simulink model "sim3el17128"  (R2019b)
settings: Solver=ode45  StartTime=0.0  StopTime=10  MaxStep=1e-4  RelTol=1e-4
values from neighbouring files (symbols this model uses):
  b1 = 0.1796    [scriptsim3el17128.m]
  b2 = 0.0012    [scriptsim3el17128.m]
  Idref = psi_hat/LM    (= 5.01212611156)    [scriptsim3el17128.m]
  Iqref = sqrt(Iref^2-Idref^2)    [scriptsim3el17128.m]
  J = 0.08    [scriptsim3el17128.m]
  K = 1/sqrt(2)    [scriptsim3el17128.m]
  Ki = alphaC*(R+Ra)    [scriptsim3el17128.m]
  kip = alphaP*alphaP/psi_hat    (= 19516.1290323)    [scriptsim3el17128.m]
  Kp = alphaC*L    [scriptsim3el17128.m]
  kpp = 2*alphaP/psi_hat    (= 354.838709677)    [scriptsim3el17128.m]
  L = Lsigma    (= 0.0227)    [scriptsim3el17128.m]
  LM = 0.1237    [scriptsim3el17128.m]
  Lsigma = 0.0227    [scriptsim3el17128.m]
  np = 2    [scriptsim3el17128.m]
  phi_a = 0    [scriptsim3el17128.m]
  phi_b = -2*pi/3    (= -2.09439510239)    [scriptsim3el17128.m]
  phi_c = -4*pi/3    (= -4.18879020479)    [scriptsim3el17128.m]
  psi_hat = 0.62    [scriptsim3el17128.m]
  Ra = alphaC*L - R    [scriptsim3el17128.m]
  refsw = 0    [scriptsim3el17128.m]
  RR = 0.8197    [scriptsim3el17128.m]
  Rs = 2.2667    [scriptsim3el17128.m]
  sw1 = 1    [scriptsim3el17128.m]
  sw2 = 1    [scriptsim3el17128.m]
  sw3 = 1    [scriptsim3el17128.m]
  tL = 26.8    [scriptsim3el17128.m]
  Vhat = 230*sqrt(2)    [scriptsim3el17128.m]
  w = 2*pi*f    (= 314.159265359)    [scriptsim3el17128.m]
undefined symbols (not defined in the file or in its folder): magnitude
settings Model: DataTypeOverride=Double  MinMaxOverflowLogging=ForceOff  Creator=user  LastModifiedBy=user
settings SolverCC: ZeroCrossAlgorithm=Adaptive
settings DebuggingCC: IgnoredZcDiagnostic=none

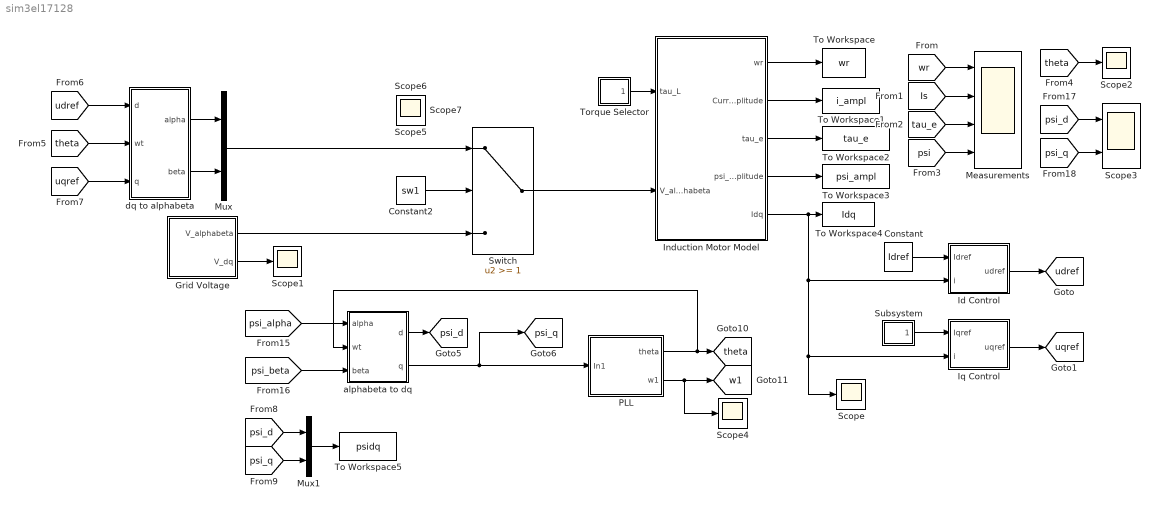
== system sim3el17128 ==
  Constant : Constant  Value=Idref
  Constant2 : Constant  Value=sw1
  Grid Voltage : Subsystem
  Id Control : Subsystem
  Induction Motor Model : Subsystem
  Iq Control : Subsystem
  Measurements : Scope  NumInputPorts=4
  Mux : Mux  Inputs=2
  Mux1 : Mux  Inputs=2
  PLL : Subsystem
  Scope{,1..2,4..7} (7 alike) : Scope
  Scope3 : Scope  NumInputPorts=2
  Subsystem : Subsystem
  Switch : Switch  Threshold=1
  To Workspace : ToWorkspace  VariableName=wr  SaveFormat=Timeseries  SampleTime=-1
  To Workspace1 : ToWorkspace  VariableName=i_ampl  SaveFormat=Timeseries  SampleTime=-1
  To Workspace2 : ToWorkspace  VariableName=tau_e  SaveFormat=Timeseries  SampleTime=-1
  To Workspace3 : ToWorkspace  VariableName=psi_ampl  SaveFormat=Timeseries  SampleTime=-1
  To Workspace4 : ToWorkspace  VariableName=Idq  SaveFormat=Timeseries  SampleTime=-1
  To Workspace5 : ToWorkspace  VariableName=psidq  SaveFormat=Timeseries  SampleTime=-1
  Torque Selector : Subsystem
  alphabeta to dq : Subsystem
  dq to alphabeta : Subsystem
  tag scope: psi_d=global, psi_q=global, theta=global, udref=global, uqref=global, w1=global
  wires:
  Induction Motor Model/1(wr) -> To Workspace/1
  Induction Motor Model/3(tau_e) -> To Workspace2/1
  Induction Motor Model/2(Current amplitude) -> To Workspace1/1
  Induction Motor Model/4(psi_amplitude) -> To Workspace3/1
  [wr] -> Measurements/1
  [Is] -> Measurements/2
  [tau_e] -> Measurements/3
  [psi] -> Measurements/4
  [theta] -> Scope2/1
  [theta] -> dq to alphabeta/2(wt)
  dq to alphabeta/1(alpha) -> Mux/1
  dq to alphabeta/2(beta) -> Mux/2
  [psi_q] -> Scope3/2
  [psi_d] -> Scope3/1
  PLL/1(theta) -> alphabeta to dq/2(wt), [theta]
  alphabeta to dq/2(q) -> [psi_q], PLL/1(In1)
  [psi_alpha] -> alphabeta to dq/1(alpha)
  PLL/2(w1) -> Scope4/1, [w1]
  [psi_beta] -> alphabeta to dq/3(beta)
  alphabeta to dq/1(d) -> [psi_d]
  [udref] -> dq to alphabeta/1(d)
  [uqref] -> dq to alphabeta/3(q)
  Induction Motor Model/5(Idq) -> To Workspace4/1, Id Control/2(i), Scope/1, Iq Control/2(i)
  Iq Control/1(uqref) -> [uqref]
  Constant/1 -> Id Control/1(Idref)
  Id Control/1(udref) -> [udref]
  Torque Selector/1(tau_L) -> Induction Motor Model/1(tau_L)
  Switch/1 -> Induction Motor Model/2(V_alphabeta)
  Grid Voltage/1(V_alphabeta) -> Switch/3
  Constant2/1 -> Switch/2
  Mux/1 -> Switch/1
  Grid Voltage/2(V_dq) -> Scope1/1
  [psi_q] -> Mux1/2
  [psi_d] -> Mux1/1
  Mux1/1 -> To Workspace5/1
  Subsystem/1(Iqref) -> Iq Control/1(Iqref)

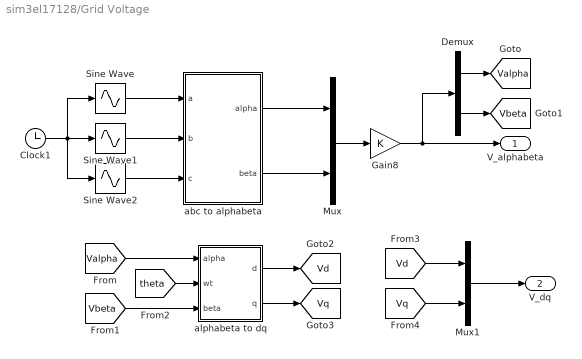
== system sim3el17128/Grid Voltage ==
  Clock1 : Clock
  Demux : Demux  Outputs=2
  Gain8 : Gain  Gain=K
  Mux : Mux  Inputs=2
  Mux1 : Mux  Inputs=2
  Sine Wave : Sin  TimeSource=Use external signal  Amplitude=Vhat  Frequency=w  Phase=phi_a  SampleTime=0
  Sine Wave1 : Sin  TimeSource=Use external signal  Amplitude=Vhat  Frequency=w  Phase=phi_b  SampleTime=0
  Sine Wave2 : Sin  TimeSource=Use external signal  Amplitude=Vhat  Frequency=w  Phase=phi_c  SampleTime=0
  abc to alphabeta : Subsystem
  alphabeta to dq : Subsystem
  V_alphabeta : Outport
  V_dq : Outport  Port=2
  tag scope: Valpha=global, Vbeta=global, Vd=global, Vq=global
  wires:
  Clock1/1 -> Sine Wave1/1, Sine Wave2/1, Sine Wave/1
  Mux/1 -> Gain8/1
  Gain8/1 -> Demux/1, V_alphabeta/1
  Demux/2 -> [Vbeta]
  Demux/1 -> [Valpha]
  [Valpha] -> alphabeta to dq/1(alpha)
  [Vbeta] -> alphabeta to dq/3(beta)
  [theta] -> alphabeta to dq/2(wt)
  alphabeta to dq/1(d) -> [Vd]
  alphabeta to dq/2(q) -> [Vq]
  [Vq] -> Mux1/2
  [Vd] -> Mux1/1
  Mux1/1 -> V_dq/1
  Sine Wave/1 -> abc to alphabeta/1(a)
  Sine Wave1/1 -> abc to alphabeta/2(b)
  Sine Wave2/1 -> abc to alphabeta/3(c)
  abc to alphabeta/1(alpha) -> Mux/1
  abc to alphabeta/2(beta) -> Mux/2

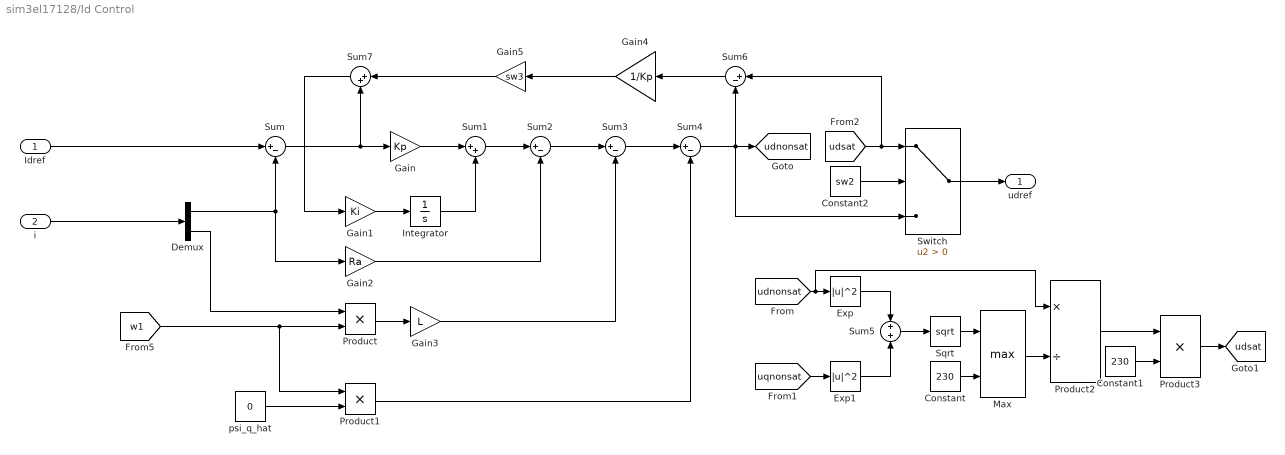
== system sim3el17128/Id Control ==
  Idref : Inport
  i : Inport  Port=2
  Constant : Constant  Value=230
  Constant1 : Constant  Value=230
  Constant2 : Constant  Value=sw2
  Demux : Demux  Outputs=2
  Exp : Math  Operator=magnitude^2  SignedPower=off  SaturateOnIntegerOverflow=on
  Exp1 : Math  Operator=magnitude^2  SignedPower=off  SaturateOnIntegerOverflow=on
  Gain : Gain  Gain=Kp
  Gain1 : Gain  Gain=Ki
  Gain2 : Gain  Gain=Ra
  Gain3 : Gain  Gain=L
  Gain4 : Gain  Gain=1/Kp
  Gain5 : Gain  Gain=sw3
  Integrator : Integrator
  Max : MinMax  Function=max  Inputs=2
  Product : Product
  Product1 : Product
  Product2 : Product  Inputs=*/
  Product3 : Product
  Sqrt : Sqrt  SaturateOnIntegerOverflow=on
  Sum{,2..4,6} (5 alike) : Sum  Inputs=|+-
  Sum1 : Sum  Inputs=|++
  Sum5 : Sum
  Sum7 : Sum  Inputs=|++
  Switch : Switch  Criteria=u2 > Threshold
  psi_q_hat : Constant  Value=0
  udref : Outport
  tag scope: udnonsat=global, udsat=global
  wires:
  Sum/1 -> Sum7/2, Gain/1
  Product1/1 -> Sum4/2
  psi_q_hat/1 -> Product1/2
  Demux/2 -> Product/1
  Sum3/1 -> Sum4/1
  Gain2/1 -> Sum2/2
  Demux/1 -> Gain2/1, Sum/2
  Gain/1 -> Sum1/1
  Sum2/1 -> Sum3/1
  Sum1/1 -> Sum2/1
  Gain3/1 -> Sum3/2
  Gain1/1 -> Integrator/1
  Product/1 -> Gain3/1
  Integrator/1 -> Sum1/2
  i/1 -> Demux/1
  Idref/1 -> Sum/1
  [udnonsat] -> Product2/1, Exp/1
  [uqnonsat] -> Exp1/1
  Exp/1 -> Sum5/1
  Exp1/1 -> Sum5/2
  Sum5/1 -> Sqrt/1
  Sqrt/1 -> Max/1
  Constant/1 -> Max/2
  Max/1 -> Product2/2
  Product2/1 -> Product3/1
  Constant1/1 -> Product3/2
  Product3/1 -> [udsat]
  [udsat] -> Switch/1, Sum6/1
  Sum7/1 -> Gain1/1
  Gain4/1 -> Gain5/1
  Sum6/1 -> Gain4/1
  [w1] -> Product1/1, Product/2
  Switch/1 -> udref/1
  Constant2/1 -> Switch/2
  Gain5/1 -> Sum7/1
  Sum4/1 -> Switch/3, Sum6/2, [udnonsat]

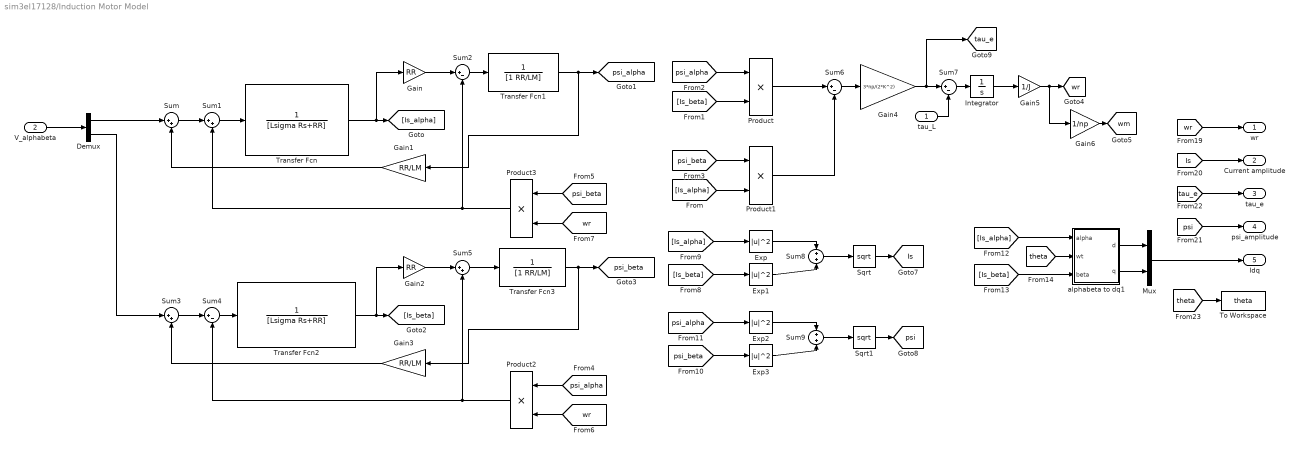
== system sim3el17128/Induction Motor Model ==
  tau_L : Inport
  V_alphabeta : Inport  Port=2
  Demux : Demux  Outputs=2
  Exp{,1..3} (4 alike) : Math  Operator=magnitude^2  SignedPower=off  SaturateOnIntegerOverflow=on
  Gain : Gain  Gain=RR
  Gain1 : Gain  Gain=RR/LM
  Gain2 : Gain  Gain=RR
  Gain3 : Gain  Gain=RR/LM
  Gain4 : Gain  Gain=3*np/(2*K^2)
  Gain5 : Gain  Gain=1/J
  Gain6 : Gain  Gain=1/np
  Integrator : Integrator
  Mux : Mux  Inputs=2
  Product{,1..3} (4 alike) : Product
  Sqrt : Sqrt  SaturateOnIntegerOverflow=on
  Sqrt1 : Sqrt  SaturateOnIntegerOverflow=on
  Sum{,1,3,5} (4 alike) : Sum  Inputs=|++
  Sum{2,4,6..7} (4 alike) : Sum  Inputs=|+-
  Sum8 : Sum  Inputs=+|+
  Sum9 : Sum  Inputs=+|+
  To Workspace : ToWorkspace  VariableName=theta  SaveFormat=Timeseries  SampleTime=-1
  Transfer Fcn : TransferFcn  Denominator=[Lsigma Rs+RR]
  Transfer Fcn1 : TransferFcn  Denominator=[1 RR/LM]
  Transfer Fcn2 : TransferFcn  Denominator=[Lsigma Rs+RR]
  Transfer Fcn3 : TransferFcn  Denominator=[1 RR/LM]
  alphabeta to dq1 : Subsystem
  wr : Outport
  Current amplitude : Outport  Port=2
  tau_e : Outport  Port=3
  psi_amplitude : Outport  Port=4
  Idq : Outport  Port=5
  tag scope: Is=global, psi=global, psi_alpha=global, psi_beta=global, tau_e=global, wm=global, wr=global
  wires:
  Transfer Fcn1/1 -> Gain1/1, [psi_alpha]
  Product3/1 -> Sum1/2, Sum2/2
  Product2/1 -> Sum4/2, Sum5/2
  [Is_beta] -> Exp1/1
  Gain5/1 -> Gain6/1, [wr]
  [Is_beta] -> Product/2
  Product/1 -> Sum6/1
  [wr] -> Product2/2
  Sqrt/1 -> [Is]
  Sum3/1 -> Sum4/1
  Transfer Fcn3/1 -> Gain3/1, [psi_beta]
  [psi_beta] -> Product1/1
  Sum5/1 -> Transfer Fcn3/1
  Transfer Fcn2/1 -> Gain2/1, [Is_beta]
  Sum1/1 -> Transfer Fcn/1
  V_alphabeta/1 -> Demux/1
  [Is_alpha] -> Product1/2
  Gain1/1 -> Sum/2
  Demux/2 -> Sum3/1
  Demux/1 -> Sum/1
  Exp/1 -> Sum8/1
  tau_L/1 -> Sum7/2
  Sum/1 -> Sum1/1
  Sum6/1 -> Gain4/1
  Gain4/1 -> [tau_e], Sum7/1
  Transfer Fcn/1 -> Gain/1, [Is_alpha]
  [psi_alpha] -> Product/1
  Sum2/1 -> Transfer Fcn1/1
  Gain3/1 -> Sum3/2
  Gain2/1 -> Sum5/1
  Sum4/1 -> Transfer Fcn2/1
  Product1/1 -> Sum6/2
  [Is_alpha] -> Exp/1
  Sum8/1 -> Sqrt/1
  Gain/1 -> Sum2/1
  [wr] -> Product3/2
  [psi_beta] -> Product3/1
  Sum7/1 -> Integrator/1
  Integrator/1 -> Gain5/1
  [psi_alpha] -> Product2/1
  Exp1/1 -> Sum8/2
  Sum9/1 -> Sqrt1/1
  [psi_alpha] -> Exp2/1
  Exp3/1 -> Sum9/2
  [psi_beta] -> Exp3/1
  Exp2/1 -> Sum9/1
  Sqrt1/1 -> [psi]
  Mux/1 -> Idq/1
  alphabeta to dq1/2(q) -> Mux/2
  alphabeta to dq1/1(d) -> Mux/1
  [Is_beta] -> alphabeta to dq1/3(beta)
  [Is_alpha] -> alphabeta to dq1/1(alpha)
  [theta] -> alphabeta to dq1/2(wt)
  [wr] -> wr/1
  [Is] -> Current amplitude/1
  [psi] -> psi_amplitude/1
  [tau_e] -> tau_e/1
  [theta] -> To Workspace/1
  Gain6/1 -> [wm]

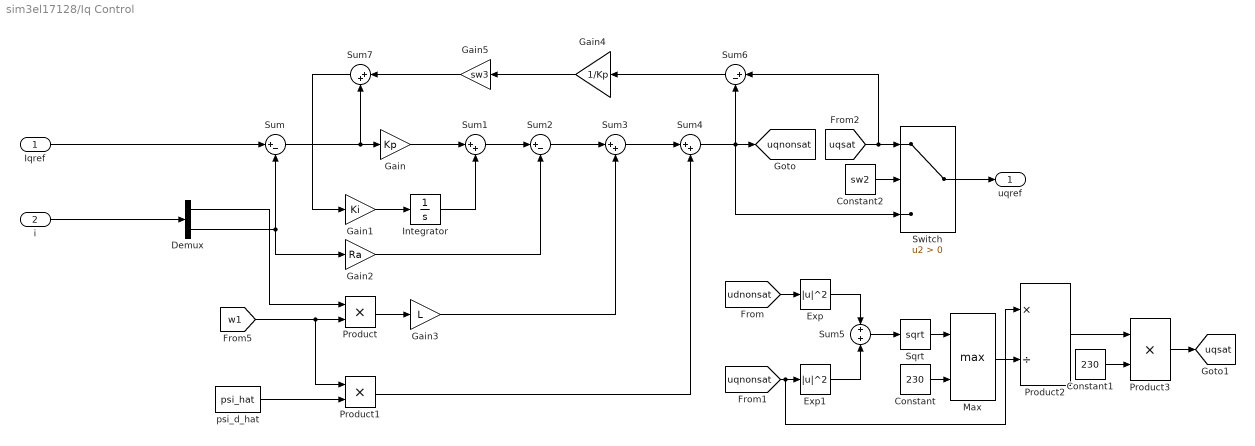
== system sim3el17128/Iq Control ==
  Iqref : Inport
  i : Inport  Port=2
  Constant : Constant  Value=230
  Constant1 : Constant  Value=230
  Constant2 : Constant  Value=sw2
  Demux : Demux  Outputs=2
  Exp : Math  Operator=magnitude^2  SignedPower=off  SaturateOnIntegerOverflow=on
  Exp1 : Math  Operator=magnitude^2  SignedPower=off  SaturateOnIntegerOverflow=on
  Gain : Gain  Gain=Kp
  Gain1 : Gain  Gain=Ki
  Gain2 : Gain  Gain=Ra
  Gain3 : Gain  Gain=L
  Gain4 : Gain  Gain=1/Kp
  Gain5 : Gain  Gain=sw3
  Integrator : Integrator
  Max : MinMax  Function=max  Inputs=2
  Product : Product
  Product1 : Product
  Product2 : Product  Inputs=*/
  Product3 : Product
  Sqrt : Sqrt  SaturateOnIntegerOverflow=on
  Sum : Sum  Inputs=|+-
  Sum{1,3..4,7} (4 alike) : Sum  Inputs=|++
  Sum2 : Sum  Inputs=|+-
  Sum5 : Sum
  Sum6 : Sum  Inputs=|+-
  Switch : Switch  Criteria=u2 > Threshold
  psi_d_hat : Constant  Value=psi_hat
  uqref : Outport
  tag scope: uqnonsat=global, uqsat=global
  wires:
  Iqref/1 -> Sum/1
  i/1 -> Demux/1
  Integrator/1 -> Sum1/2
  Product/1 -> Gain3/1
  Gain1/1 -> Integrator/1
  Gain3/1 -> Sum3/2
  Sum1/1 -> Sum2/1
  Sum2/1 -> Sum3/1
  Gain/1 -> Sum1/1
  Gain2/1 -> Sum2/2
  Sum3/1 -> Sum4/1
  psi_d_hat/1 -> Product1/2
  Product1/1 -> Sum4/2
  [w1] -> Product/2, Product1/1
  Demux/2 -> Sum/2, Gain2/1
  Demux/1 -> Product/1
  Sum/1 -> Sum7/2, Gain/1
  Exp1/1 -> Sum5/2
  Constant1/1 -> Product3/2
  Max/1 -> Product2/2
  Sum5/1 -> Sqrt/1
  Constant/1 -> Max/2
  Product3/1 -> [uqsat]
  Sqrt/1 -> Max/1
  Product2/1 -> Product3/1
  [uqnonsat] -> Product2/1, Exp1/1
  Exp/1 -> Sum5/1
  [udnonsat] -> Exp/1
  Sum6/1 -> Gain4/1
  Gain4/1 -> Gain5/1
  Sum7/1 -> Gain1/1
  [uqsat] -> Sum6/1, Switch/1
  Switch/1 -> uqref/1
  Constant2/1 -> Switch/2
  Gain5/1 -> Sum7/1
  Sum4/1 -> Switch/3, Sum6/2, [uqnonsat]

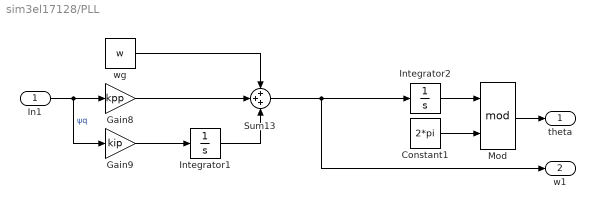
== system sim3el17128/PLL ==
  In1 : Inport
  Constant1 : Constant  Value=2*pi
  Gain8 : Gain  Gain=kpp
  Gain9 : Gain  Gain=kip
  Integrator1 : Integrator
  Integrator2 : Integrator
  Mod : Math  Operator=mod  SignedPower=off  SaturateOnIntegerOverflow=on
  Sum13 : Sum  Inputs=+++
  wg : Constant  Value=w
  theta : Outport
  w1 : Outport  Port=2
  wires:
  In1/1 -> Gain9/1, Gain8/1  "ψq"
  Constant1/1 -> Mod/2
  Gain8/1 -> Sum13/2
  wg/1 -> Sum13/1
  Gain9/1 -> Integrator1/1
  Integrator1/1 -> Sum13/3
  Sum13/1 -> w1/1, Integrator2/1
  Mod/1 -> theta/1
  Integrator2/1 -> Mod/1

== system sim3el17128/Subsystem ==
  Constant1 : Constant  Value=Iqref
  Constant2 : Constant  Value=0
  Constant3 : Constant  Value=refsw
  Constant4 : Constant  Value=Iqref
  Switch1 : Switch  Threshold=w
  Switch2 : Switch  Criteria=u2 > Threshold
  Iqref : Outport
  wires:
  Constant2/1 -> Switch1/1
  Constant1/1 -> Switch1/3
  [wr] -> Switch1/2
  Switch1/1 -> Switch2/1
  Constant4/1 -> Switch2/3
  Switch2/1 -> Iqref/1
  Constant3/1 -> Switch2/2

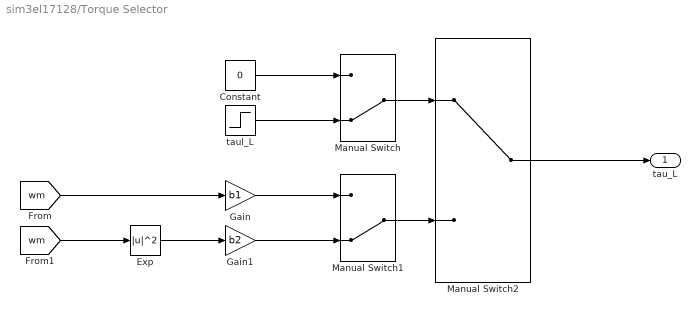
== system sim3el17128/Torque Selector ==
  Constant : Constant  Value=0
  Exp : Math  Operator=magnitude^2  SignedPower=off  SaturateOnIntegerOverflow=on
  Gain : Gain  Gain=b1
  Gain1 : Gain  Gain=b2
  Manual Switch : ManualSwitch  CurrentSetting=0
  Manual Switch1 : ManualSwitch  CurrentSetting=0
  Manual Switch2 : ManualSwitch
  taul_L : Step  Time=5  After=tL  SampleTime=0
  tau_L : Outport
  wires:
  [wm] -> Gain/1
  Gain1/1 -> Manual Switch1/2
  taul_L/1 -> Manual Switch/2
  Exp/1 -> Gain1/1
  [wm] -> Exp/1
  Constant/1 -> Manual Switch/1
  Gain/1 -> Manual Switch1/1
  Manual Switch2/1 -> tau_L/1
  Manual Switch1/1 -> Manual Switch2/2
  Manual Switch/1 -> Manual Switch2/1

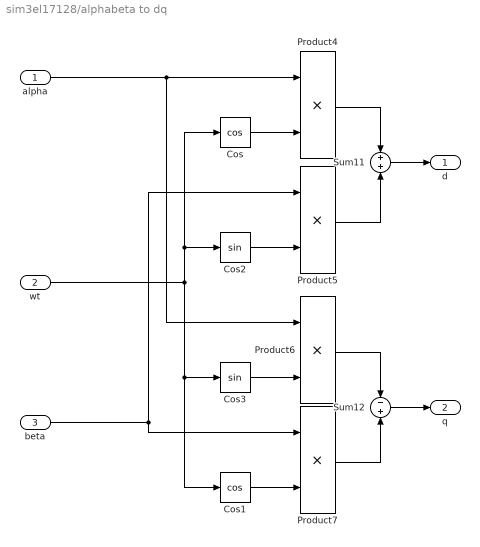
== system sim3el17128/alphabeta to dq ==
  alpha : Inport
  wt : Inport  Port=2
  beta : Inport  Port=3
  Cos : Trigonometry  Operator=cos
  Cos1 : Trigonometry  Operator=cos
  Cos2 : Trigonometry
  Cos3 : Trigonometry
  Product{4..7} (4 alike) : Product
  Sum11 : Sum
  Sum12 : Sum  Inputs=-+
  d : Outport
  q : Outport  Port=2
  wires:
  Cos3/1 -> Product6/2
  Product6/1 -> Sum12/1
  Sum11/1 -> d/1
  alpha/1 -> Product4/1, Product6/1
  wt/1 -> Cos3/1, Cos1/1, Cos2/1, Cos/1
  Product4/1 -> Sum11/1
  beta/1 -> Product7/1, Product5/1
  Product7/1 -> Sum12/2
  Cos1/1 -> Product7/2
  Product5/1 -> Sum11/2
  Cos/1 -> Product4/2
  Cos2/1 -> Product5/2
  Sum12/1 -> q/1

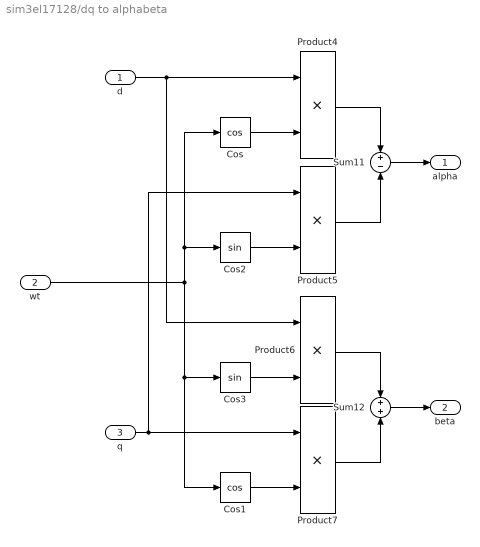
== system sim3el17128/dq to alphabeta ==
  d : Inport
  wt : Inport  Port=2
  q : Inport  Port=3
  Cos : Trigonometry  Operator=cos
  Cos1 : Trigonometry  Operator=cos
  Cos2 : Trigonometry
  Cos3 : Trigonometry
  Product{4..7} (4 alike) : Product
  Sum11 : Sum  Inputs=+-
  Sum12 : Sum
  alpha : Outport
  beta : Outport  Port=2
  wires:
  Cos3/1 -> Product6/2
  Product6/1 -> Sum12/1
  Sum11/1 -> alpha/1
  d/1 -> Product4/1, Product6/1
  wt/1 -> Cos3/1, Cos1/1, Cos2/1, Cos/1
  Product4/1 -> Sum11/1
  q/1 -> Product5/1, Product7/1
  Product7/1 -> Sum12/2
  Cos1/1 -> Product7/2
  Product5/1 -> Sum11/2
  Cos/1 -> Product4/2
  Cos2/1 -> Product5/2
  Sum12/1 -> beta/1

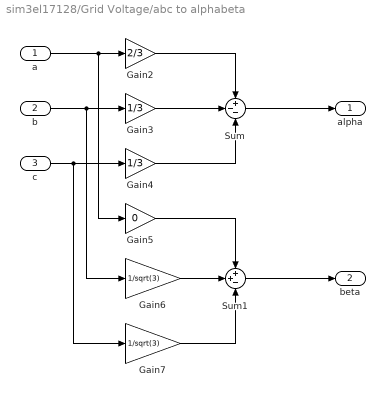
== system sim3el17128/Grid Voltage/abc to alphabeta ==
  a : Inport
  b : Inport  Port=2
  c : Inport  Port=3
  Gain2 : Gain  Gain=2/3
  Gain3 : Gain  Gain=1/3
  Gain4 : Gain  Gain=1/3
  Gain5 : Gain  Gain=0
  Gain6 : Gain  Gain=1/sqrt(3)
  Gain7 : Gain  Gain=1/sqrt(3)
  Sum : Sum  Inputs=+--
  Sum1 : Sum  Inputs=++-
  alpha : Outport
  beta : Outport  Port=2
  wires:
  Gain4/1 -> Sum/3
  Gain3/1 -> Sum/2
  a/1 -> Gain5/1, Gain2/1
  Gain6/1 -> Sum1/2
  c/1 -> Gain7/1, Gain4/1
  Gain7/1 -> Sum1/3
  Gain5/1 -> Sum1/1
  Gain2/1 -> Sum/1
  b/1 -> Gain6/1, Gain3/1
  Sum/1 -> alpha/1
  Sum1/1 -> beta/1

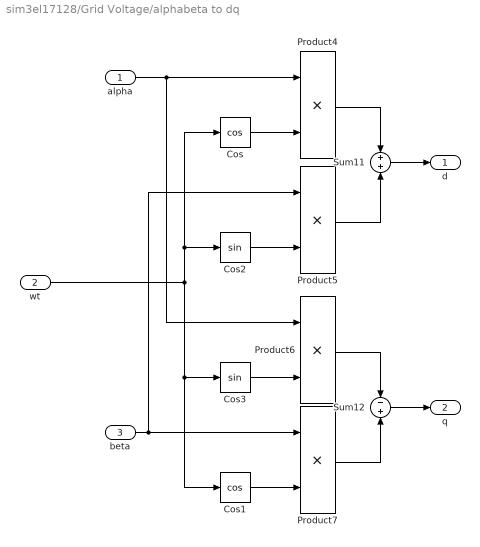
== system sim3el17128/Grid Voltage/alphabeta to dq ==
  alpha : Inport
  wt : Inport  Port=2
  beta : Inport  Port=3
  Cos : Trigonometry  Operator=cos
  Cos1 : Trigonometry  Operator=cos
  Cos2 : Trigonometry
  Cos3 : Trigonometry
  Product{4..7} (4 alike) : Product
  Sum11 : Sum
  Sum12 : Sum  Inputs=-+
  d : Outport
  q : Outport  Port=2
  wires:
  Cos3/1 -> Product6/2
  Product6/1 -> Sum12/1
  Sum11/1 -> d/1
  alpha/1 -> Product4/1, Product6/1
  wt/1 -> Cos3/1, Cos1/1, Cos2/1, Cos/1
  Product4/1 -> Sum11/1
  beta/1 -> Product5/1, Product7/1
  Product7/1 -> Sum12/2
  Cos1/1 -> Product7/2
  Product5/1 -> Sum11/2
  Cos/1 -> Product4/2
  Cos2/1 -> Product5/2
  Sum12/1 -> q/1

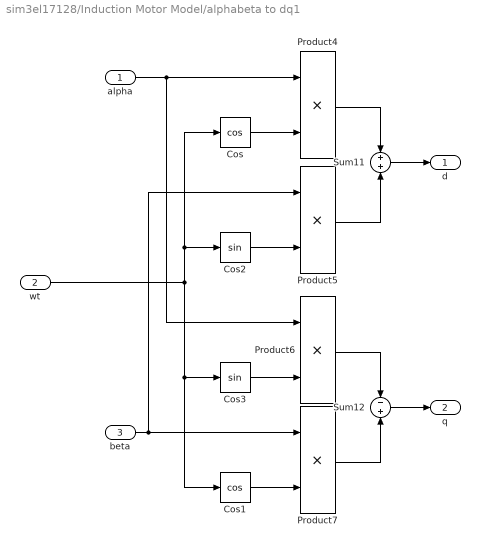
== system sim3el17128/Induction Motor Model/alphabeta to dq1 ==
  alpha : Inport
  wt : Inport  Port=2
  beta : Inport  Port=3
  Cos : Trigonometry  Operator=cos
  Cos1 : Trigonometry  Operator=cos
  Cos2 : Trigonometry
  Cos3 : Trigonometry
  Product{4..7} (4 alike) : Product
  Sum11 : Sum
  Sum12 : Sum  Inputs=-+
  d : Outport
  q : Outport  Port=2
  wires:
  Sum12/1 -> q/1
  Cos2/1 -> Product5/2
  Cos/1 -> Product4/2
  Product5/1 -> Sum11/2
  Cos1/1 -> Product7/2
  Product7/1 -> Sum12/2
  beta/1 -> Product7/1, Product5/1
  Product4/1 -> Sum11/1
  wt/1 -> Cos/1, Cos2/1, Cos1/1, Cos3/1
  alpha/1 -> Product6/1, Product4/1
  Sum11/1 -> d/1
  Product6/1 -> Sum12/1
  Cos3/1 -> Product6/2
